simulink model "P14_24"  (R2016a)
settings: Solver=VariableStepAuto  StartTime=0.0  StopTime=10.0  RelTol=1e-3
settings Model: Creator=lenovo  LastModifiedBy=lenovo

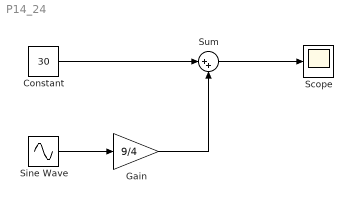
== system P14_24 ==
  Constant : Constant  Value=30
  Gain : Gain  Gain=9/4
  Scope : Scope
  Sine Wave : Sin  Amplitude=10  SampleTime=0
  Sum : Sum  Inputs=|++
  wires:
  Sum/1 -> Scope/1
  Constant/1 -> Sum/1
  Sine Wave/1 -> Gain/1
  Gain/1 -> Sum/2
